simulink model "sdbe_8_11"  (R2012b)
settings: Solver=VariableStepDiscrete  SolverMode=SingleTasking  StartTime=0.0  StopTime=10000  RelTol=1e-3
PreLoadFcn:
  | counter_vals
undefined symbols (not defined in the file or in its folder): sfp
libraries: xbsIndex_r4 x6687, casper_library_misc x35, casper_library_delays x27, dspsigops x16, xps_library x10, r2dbe_vdif_lib x4, r2dbe_adc_lib x3, simulink x1
(part 19 of 58)

== system sdbe_8_11/get_data_from_pkt1/scope ==
  data : Inport
  valid : Inport  Port=2
  Constant : xbsIndex_r4/Constant  const=2  gui_display_data_type=Fixed-point  arith_type=Unsigned  n_bits=7  bin_pt=0  preci_type=Single  exp_width=8  frac_width=24  explicit_period=on  period=1  equ=P=C  opselect=C  inp2=PCIN>>17  opr=+  inp1=P  carry=CIN  dbl_ovrd=off  block_type=constant
  Delay : xbsIndex_r4/Delay  rst=off  infoeditControl=Selection of Reset will increase slice count due to use of real FFs and instead of SRLs  en=off  latency=3  dbl_ovrd=off  reg_retiming=off  block_type=delay
  Delay1 : xbsIndex_r4/Delay  rst=off  infoeditControl=Selection of Reset will increase slice count due to use of real FFs and instead of SRLs  en=off  latency=3  dbl_ovrd=off  reg_retiming=off  block_type=delay
  Disregard Subsystem : xbsIndex_r4/Disregard Subsystem  Tag=discardX  block_type=disregard
  Gateway Out{1..6} (6 alike) : xbsIndex_r4/Gateway Out  inherit_from_input=off  hdl_port=on  timing_constraint=None  locs_specified=off  LOCs={}  UseAsDAC=off  DACChannel='1'  block_type=gatewayout
  Mux : Mux  Inputs=6
  Scope : Scope
      settings: SaveName=ScopeData8
  bus_expand1 : Subsystem  AncestorBlock=casper_library_flow_control/bus_expand  mask(bus_expand){mode=divisions of equal size, outputNum=16, outputWidth=4, outputBinaryPt=0, outputArithmeticType=1, show_format=off, outputToWorkspace=off, variablePrefix=out, outputToModelAsWell=on}
      mask prompts: outputNum "Number of outputs:"; outputWidth "Output width:"; outputBinaryPt "Output binary point position:"; outputArithmeticType "Output arithmetic type (ufix=0, fix=1, bool=2):"; show_format "Print format string?"; outputToWorkspace "Output to workspace?"; variablePrefix "Variable name prefix:"; outputToModelAsWell "Output to model as well?"
      mask help:
      | Expands a 'bus' made using a bus_create or Xilinx
      | concat block.
      | The input will be divided into the specified number
      | of outputs with the specified arithmetic types.
      | Divisions are made from most significant bit.
      mask init: same as sdbe_8_11/get_data_from_pkt/scope/bus_expand1
      settings: AttributesFormatString=16 outputs
      mask TypeOptions mode: divisions of equal size | divisions of arbitrary size
      mask Callback mode: bus_expand_callback();
      mask Callback outputWidth: bus_expand_callback();
      mask Callback outputToWorkspace: bus_expand_callback();
  quant0 : Subsystem
  quant1 : Subsystem
  quant10 : Subsystem
  quant11 : Subsystem
  quant12 : Subsystem
  quant13 : Subsystem
  quant14 : Subsystem
  quant15 : Subsystem
  quant2 : Subsystem
  quant3 : Subsystem
  quant4 : Subsystem
  quant5 : Subsystem
  quant6 : Subsystem
  quant7 : Subsystem
  quant8 : Subsystem
  quant9 : Subsystem
  wires:
  Delay1/1 -> Gateway Out5/1
  Delay/1 -> Gateway Out6/1
  Mux/1 -> Scope/1
  Gateway Out6/1 -> Mux/6
  valid/1 -> Delay/1
  Gateway Out4/1 -> Mux/5
  [p0r_ch3] -> Gateway Out4/1
  Gateway Out3/1 -> Mux/4
  [p0r_ch2] -> Gateway Out3/1
  Gateway Out2/1 -> Mux/3
  [p0r_ch1] -> Gateway Out2/1
  [p0r_ch0] -> Gateway Out1/1
  [p0r_ch0_before] -> Delay1/1
  bus_expand1/7(out10) -> quant6/1(din4)
  bus_expand1/15(out2) -> quant14/1(din4)
  bus_expand1/8(out9) -> quant7/1(din4)
  bus_expand1/13(out4) -> quant12/1(din4)
  bus_expand1/4(out13) -> quant3/1(din4)
  bus_expand1/12(out5) -> quant11/1(din4)
  bus_expand1/10(out7) -> quant9/1(din4)
  bus_expand1/3(out14) -> quant2/1(din4)
  bus_expand1/5(out12) -> quant4/1(din4)
  bus_expand1/1(msb_out16) -> quant0/1(din4), [p0r_ch0_before]
  bus_expand1/11(out6) -> quant10/1(din4)
  bus_expand1/2(out15) -> quant1/1(din4)
  bus_expand1/16(lsb_out1) -> quant15/1(din4)
  bus_expand1/6(out11) -> quant5/1(din4)
  bus_expand1/14(out3) -> quant13/1(din4)
  bus_expand1/9(out8) -> quant8/1(din4)
  Constant/1 -> quant0/2(thr), quant1/2(thr), quant2/2(thr), quant3/2(thr), quant4/2(thr), quant5/2(thr), quant6/2(thr), quant7/2(thr), quant8/2(thr), quant9/2(thr), quant10/2(thr), quant11/2(thr), quant12/2(thr), quant13/2(thr), quant14/2(thr), quant15/2(thr)
  quant0/1(dout2) -> [p0r_ch0]
  quant1/1(dout2) -> [p0i_ch0]
  quant3/1(dout2) -> [p1i_ch0]
  quant2/1(dout2) -> [p1r_ch0]
  quant6/1(dout2) -> [p1r_ch1]
  quant7/1(dout2) -> [p1i_ch1]
  quant4/1(dout2) -> [p0r_ch1]
  quant5/1(dout2) -> [p0i_ch1]
  quant13/1(dout2) -> [p0i_ch3]
  quant14/1(dout2) -> [p1r_ch3]
  quant9/1(dout2) -> [p0i_ch2]
  quant12/1(dout2) -> [p0r_ch3]
  quant11/1(dout2) -> [p1i_ch2]
  quant8/1(dout2) -> [p0r_ch2]
  quant15/1(dout2) -> [p1i_ch3]
  quant10/1(dout2) -> [p1r_ch2]
  Gateway Out1/1 -> Mux/2
  Gateway Out5/1 -> Mux/1
  data/1 -> bus_expand1/1(bus_in)

== system sdbe_8_11/get_data_from_pkt2/gen_valids1 ==
  note: 1 when hdr_val is no and pkt_val is yes
  note: after eof, next high value is hdr
  note: initial value is 0
      |
      | enable on eof
      | send pkt_val through,
      | posedge on output gives hdr_val
      | hdr_val resets to get 0 again, so output is zero
  note: no lat
  note: one lat
  pkt_val : Inport
  eof : Inport  Port=2
  Constant : xbsIndex_r4/Constant  const=1  gui_display_data_type=Boolean  arith_type=Boolean  n_bits=16  bin_pt=14  preci_type=Single  exp_width=8  frac_width=24  explicit_period=off  period=1  equ=P=C  opselect=C  inp2=PCIN>>17  opr=+  inp1=P  carry=CIN  dbl_ovrd=off  block_type=constant
  Constant1 : xbsIndex_r4/Constant  const=1  gui_display_data_type=Boolean  arith_type=Boolean  n_bits=16  bin_pt=14  preci_type=Single  exp_width=8  frac_width=24  explicit_period=off  period=1  equ=P=C  opselect=C  inp2=PCIN>>17  opr=+  inp1=P  carry=CIN  dbl_ovrd=off  block_type=constant
  Delay1 : xbsIndex_r4/Delay  rst=off  infoeditControl=Selection of Reset will increase slice count due to use of real FFs and instead of SRLs  en=off  latency=1  dbl_ovrd=off  reg_retiming=off  block_type=delay
  Delay2 : xbsIndex_r4/Delay  rst=off  infoeditControl=Selection of Reset will increase slice count due to use of real FFs and instead of SRLs  en=off  latency=1  dbl_ovrd=off  reg_retiming=off  block_type=delay
  Logical : xbsIndex_r4/Logical  logical_function=XOR  inputs=2  en=off  latency=0  precision=Full  arith_type=Unsigned  n_bits=16  bin_pt=0  align_bp=on  dbl_ovrd=off  block_type=logical
  Logical1 : xbsIndex_r4/Logical  logical_function=AND  inputs=2  en=off  latency=0  precision=Full  arith_type=Unsigned  n_bits=16  bin_pt=0  align_bp=on  dbl_ovrd=off  block_type=logical
  Register : xbsIndex_r4/Register  init=0  rst=on  en=on  dbl_ovrd=off  block_type=register
  Register1 : xbsIndex_r4/Register  init=0  rst=on  en=on  dbl_ovrd=off  block_type=register
  Register2 : xbsIndex_r4/Register  init=0  rst=off  en=on  dbl_ovrd=off  block_type=register
  posedge : casper_library_misc/posedge  Tag=Rising Edge Detector
  hdr_val : Outport
  data_val : Outport  Port=2
  wires:
  [hdr_val] -> Register1/2
  Constant/1 -> Register1/1
  [hdr_val] -> Register/2
  [pkt_val] -> Delay1/1
  Register1/1 -> Register/3
  pkt_val/1 -> Register/1, [pkt_val]
  eof/1 -> Register2/2, Register1/3
  Register/1 -> posedge/1
  posedge/1 -> Logical/1, hdr_val/1, [hdr_val]
  Logical/1 -> data_val/1
  Logical1/1 -> Logical/2
  Delay1/1 -> Logical1/1
  Constant1/1 -> Register2/1
  Register2/1 -> Delay2/1
  Delay2/1 -> Logical1/2

== system sdbe_8_11/get_data_from_pkt2/npkts ==
  out_reg : Inport
  assert_reg : xbsIndex_r4/Assert  assert_type=on  type_source=Explicitly  gui_display_data_type=Fixed-point  arith_type=Unsigned  n_bits=32  bin_pt=0  preci_type=Single  exp_width=8  frac_width=24  assert_rate=off  rate_source=Explicitly  period=1  output_port=on  block_type=assert
  cast_gw : xbsIndex_r4/Convert  gui_display_data_type=Fixed-point  arith_type=Unsigned  n_bits=32  bin_pt=0  float_type=Single  exp_bits=8  fraction_bits=24  quantization=Truncate  overflow=Wrap  en=off  latency=0  dbl_ovrd=off  pipeline=off  block_type=convert
  io_delay : xbsIndex_r4/Delay  rst=off  infoeditControl=Selection of Reset will increase slice count due to use of real FFs and instead of SRLs  en=off  latency=0  dbl_ovrd=off  reg_retiming=on  block_type=delay
  reint1 : xbsIndex_r4/Reinterpret  force_arith_type=on  arith_type=Unsigned  force_bin_pt=on  bin_pt=0  block_type=reinterpret
  sdbe_8_11_get_data_from_pkt2_npkts_user_data_in : xbsIndex_r4/Gateway Out  inherit_from_input=off  hdl_port=on  timing_constraint=None  locs_specified=off  LOCs={}  UseAsDAC=off  DACChannel='1'  block_type=gatewayout
  sim_out : Outport
  wires:
  io_delay/1 -> cast_gw/1
  cast_gw/1 -> sdbe_8_11_get_data_from_pkt2_npkts_user_data_in/1
  sdbe_8_11_get_data_from_pkt2_npkts_user_data_in/1 -> sim_out/1
  out_reg/1 -> assert_reg/1
  assert_reg/1 -> reint1/1
  reint1/1 -> io_delay/1

== system sdbe_8_11/get_data_from_pkt2/rst ==
  sim_1 : Inport
  io_delay : xbsIndex_r4/Delay  rst=off  infoeditControl=Selection of Reset will increase slice count due to use of real FFs and instead of SRLs  en=off  latency=0  dbl_ovrd=off  reg_retiming=on  block_type=delay
  reint1 : xbsIndex_r4/Reinterpret  force_arith_type=on  arith_type=Unsigned  force_bin_pt=on  bin_pt=0  block_type=reinterpret
  sdbe_8_11_get_data_from_pkt2_rst_user_data_out : xbsIndex_r4/Gateway In  gui_display_data_type=Fixed-point  arith_type=Unsigned  n_bits=32  bin_pt=0  preci_type=Single  exp_width=8  frac_width=24  quantization="Round  (unbiased: +/- Inf)"  overflow=Saturate  period=1  dbl_ovrd=off  timing_constraint=None  locs_specified=off  LOCs={}  UseAsADC=off  ADCChannel='1'  inherit_from_input=off  hdl_port=on  block_type=gatewayin
  slice_reg : xbsIndex_r4/Slice  nbits=32  boolean_output=off  mode=Lower Bit Location + Width  bit1=0  base1=MSB of Input  bit0=0  base0=LSB of Input  dbl_ovrd=off  block_type=slice
  in_reg : Outport
  wires:
  sdbe_8_11_get_data_from_pkt2_rst_user_data_out/1 -> io_delay/1
  sim_1/1 -> sdbe_8_11_get_data_from_pkt2_rst_user_data_out/1
  io_delay/1 -> slice_reg/1
  slice_reg/1 -> reint1/1
  reint1/1 -> in_reg/1

== system sdbe_8_11/get_data_from_pkt2/rx_output ==
  sig : Inport
  val : Inport  Port=2
  eof : Inport  Port=3
  Disregard Subsystem : xbsIndex_r4/Disregard Subsystem  Tag=discardX  block_type=disregard
  Gateway Out : xbsIndex_r4/Gateway Out  inherit_from_input=off  hdl_port=on  timing_constraint=None  locs_specified=off  LOCs={}  UseAsDAC=off  DACChannel='1'  block_type=gatewayout
  Gateway Out1 : xbsIndex_r4/Gateway Out  inherit_from_input=off  hdl_port=on  timing_constraint=None  locs_specified=off  LOCs={}  UseAsDAC=off  DACChannel='1'  block_type=gatewayout
  Gateway Out2 : xbsIndex_r4/Gateway Out  inherit_from_input=off  hdl_port=on  timing_constraint=None  locs_specified=off  LOCs={}  UseAsDAC=off  DACChannel='1'  block_type=gatewayout
  Mux : Mux  Inputs=2
  Scope : Scope  NumInputPorts=2
      settings: YMin=-5~-5  YMax=5~5  SaveName=ScopeData5
  wires:
  sig/1 -> Gateway Out/1
  Gateway Out/1 -> Scope/1  "sig"
  val/1 -> Gateway Out1/1
  eof/1 -> Gateway Out2/1
  Gateway Out2/1 -> Mux/2  "eof"
  Mux/1 -> Scope/2
  Gateway Out1/1 -> Mux/1  "val"

== system sdbe_8_11/get_data_from_pkt2/rx_output1 ==
  hdr : Inport
  hdr_val : Inport  Port=2
  data : Inport  Port=3
  data_val : Inport  Port=4
  Disregard Subsystem : xbsIndex_r4/Disregard Subsystem  Tag=discardX  block_type=disregard
  Gateway Out{,1..3} (4 alike) : xbsIndex_r4/Gateway Out  inherit_from_input=off  hdl_port=on  timing_constraint=None  locs_specified=off  LOCs={}  UseAsDAC=off  DACChannel='1'  block_type=gatewayout
  Mux : Mux  Inputs=2
  Mux1 : Mux  Inputs=2
  Scope : Scope  NumInputPorts=2
      settings: YMin=0~-5  YMax=2.5e+18~5  SaveName=ScopeData5
  wires:
  Mux/1 -> Scope/2  "hdr_val_yellow_data_val_pink"
  data/1 -> Gateway Out2/1
  hdr_val/1 -> Gateway Out1/1
  hdr/1 -> Gateway Out/1
  data_val/1 -> Gateway Out3/1
  Gateway Out3/1 -> Mux/2
  Mux1/1 -> Scope/1  "hdr_yellow_data_pink"
  Gateway Out/1 -> Mux1/1  "sig"
  Gateway Out1/1 -> Mux/1  "val"
  Gateway Out2/1 -> Mux1/2  "eof"

== system sdbe_8_11/get_data_from_pkt2/scope ==
  data : Inport
  valid : Inport  Port=2
  Constant : xbsIndex_r4/Constant  const=2  gui_display_data_type=Fixed-point  arith_type=Unsigned  n_bits=7  bin_pt=0  preci_type=Single  exp_width=8  frac_width=24  explicit_period=on  period=1  equ=P=C  opselect=C  inp2=PCIN>>17  opr=+  inp1=P  carry=CIN  dbl_ovrd=off  block_type=constant
  Delay : xbsIndex_r4/Delay  rst=off  infoeditControl=Selection of Reset will increase slice count due to use of real FFs and instead of SRLs  en=off  latency=3  dbl_ovrd=off  reg_retiming=off  block_type=delay
  Delay1 : xbsIndex_r4/Delay  rst=off  infoeditControl=Selection of Reset will increase slice count due to use of real FFs and instead of SRLs  en=off  latency=3  dbl_ovrd=off  reg_retiming=off  block_type=delay
  Disregard Subsystem : xbsIndex_r4/Disregard Subsystem  Tag=discardX  block_type=disregard
  Gateway Out{1..6} (6 alike) : xbsIndex_r4/Gateway Out  inherit_from_input=off  hdl_port=on  timing_constraint=None  locs_specified=off  LOCs={}  UseAsDAC=off  DACChannel='1'  block_type=gatewayout
  Mux : Mux  Inputs=6
  Scope : Scope
      settings: SaveName=ScopeData8
  bus_expand1 : Subsystem  AncestorBlock=casper_library_flow_control/bus_expand  mask(bus_expand){mode=divisions of equal size, outputNum=16, outputWidth=4, outputBinaryPt=0, outputArithmeticType=1, show_format=off, outputToWorkspace=off, variablePrefix=out, outputToModelAsWell=on}
      mask prompts: outputNum "Number of outputs:"; outputWidth "Output width:"; outputBinaryPt "Output binary point position:"; outputArithmeticType "Output arithmetic type (ufix=0, fix=1, bool=2):"; show_format "Print format string?"; outputToWorkspace "Output to workspace?"; variablePrefix "Variable name prefix:"; outputToModelAsWell "Output to model as well?"
      mask help:
      | Expands a 'bus' made using a bus_create or Xilinx
      | concat block.
      | The input will be divided into the specified number
      | of outputs with the specified arithmetic types.
      | Divisions are made from most significant bit.
      mask init: same as sdbe_8_11/get_data_from_pkt/scope/bus_expand1
      settings: AttributesFormatString=16 outputs
      mask TypeOptions mode: divisions of equal size | divisions of arbitrary size
      mask Callback mode: bus_expand_callback();
      mask Callback outputWidth: bus_expand_callback();
      mask Callback outputToWorkspace: bus_expand_callback();
  quant0 : Subsystem
  quant1 : Subsystem
  quant10 : Subsystem
  quant11 : Subsystem
  quant12 : Subsystem
  quant13 : Subsystem
  quant14 : Subsystem
  quant15 : Subsystem
  quant2 : Subsystem
  quant3 : Subsystem
  quant4 : Subsystem
  quant5 : Subsystem
  quant6 : Subsystem
  quant7 : Subsystem
  quant8 : Subsystem
  quant9 : Subsystem
  wires:
  data/1 -> bus_expand1/1(bus_in)
  Gateway Out5/1 -> Mux/1
  Gateway Out1/1 -> Mux/2
  quant10/1(dout2) -> [p1r_ch2]
  quant15/1(dout2) -> [p1i_ch3]
  quant8/1(dout2) -> [p0r_ch2]
  quant11/1(dout2) -> [p1i_ch2]
  quant12/1(dout2) -> [p0r_ch3]
  quant9/1(dout2) -> [p0i_ch2]
  quant14/1(dout2) -> [p1r_ch3]
  quant13/1(dout2) -> [p0i_ch3]
  quant5/1(dout2) -> [p0i_ch1]
  quant4/1(dout2) -> [p0r_ch1]
  quant7/1(dout2) -> [p1i_ch1]
  quant6/1(dout2) -> [p1r_ch1]
  quant2/1(dout2) -> [p1r_ch0]
  quant3/1(dout2) -> [p1i_ch0]
  quant1/1(dout2) -> [p0i_ch0]
  quant0/1(dout2) -> [p0r_ch0]
  Constant/1 -> quant15/2(thr), quant14/2(thr), quant13/2(thr), quant12/2(thr), quant11/2(thr), quant10/2(thr), quant9/2(thr), quant8/2(thr), quant7/2(thr), quant6/2(thr), quant5/2(thr), quant4/2(thr), quant3/2(thr), quant2/2(thr), quant1/2(thr), quant0/2(thr)
  bus_expand1/9(out8) -> quant8/1(din4)
  bus_expand1/14(out3) -> quant13/1(din4)
  bus_expand1/6(out11) -> quant5/1(din4)
  bus_expand1/16(lsb_out1) -> quant15/1(din4)
  bus_expand1/2(out15) -> quant1/1(din4)
  bus_expand1/11(out6) -> quant10/1(din4)
  bus_expand1/1(msb_out16) -> [p0r_ch0_before], quant0/1(din4)
  bus_expand1/5(out12) -> quant4/1(din4)
  bus_expand1/3(out14) -> quant2/1(din4)
  bus_expand1/10(out7) -> quant9/1(din4)
  bus_expand1/12(out5) -> quant11/1(din4)
  bus_expand1/4(out13) -> quant3/1(din4)
  bus_expand1/13(out4) -> quant12/1(din4)
  bus_expand1/8(out9) -> quant7/1(din4)
  bus_expand1/15(out2) -> quant14/1(din4)
  bus_expand1/7(out10) -> quant6/1(din4)
  [p0r_ch0_before] -> Delay1/1
  [p0r_ch0] -> Gateway Out1/1
  [p0r_ch1] -> Gateway Out2/1
  Gateway Out2/1 -> Mux/3
  [p0r_ch2] -> Gateway Out3/1
  Gateway Out3/1 -> Mux/4
  [p0r_ch3] -> Gateway Out4/1
  Gateway Out4/1 -> Mux/5
  valid/1 -> Delay/1
  Gateway Out6/1 -> Mux/6
  Mux/1 -> Scope/1
  Delay/1 -> Gateway Out6/1
  Delay1/1 -> Gateway Out5/1

== system sdbe_8_11/get_data_from_pkt3/gen_valids1 ==
  note: one lat
  note: no lat
  note: initial value is 0
      |
      | enable on eof
      | send pkt_val through,
      | posedge on output gives hdr_val
      | hdr_val resets to get 0 again, so output is zero
  note: after eof, next high value is hdr
  note: 1 when hdr_val is no and pkt_val is yes
  pkt_val : Inport
  eof : Inport  Port=2
  Constant : xbsIndex_r4/Constant  const=1  gui_display_data_type=Boolean  arith_type=Boolean  n_bits=16  bin_pt=14  preci_type=Single  exp_width=8  frac_width=24  explicit_period=off  period=1  equ=P=C  opselect=C  inp2=PCIN>>17  opr=+  inp1=P  carry=CIN  dbl_ovrd=off  block_type=constant
  Constant1 : xbsIndex_r4/Constant  const=1  gui_display_data_type=Boolean  arith_type=Boolean  n_bits=16  bin_pt=14  preci_type=Single  exp_width=8  frac_width=24  explicit_period=off  period=1  equ=P=C  opselect=C  inp2=PCIN>>17  opr=+  inp1=P  carry=CIN  dbl_ovrd=off  block_type=constant
  Delay1 : xbsIndex_r4/Delay  rst=off  infoeditControl=Selection of Reset will increase slice count due to use of real FFs and instead of SRLs  en=off  latency=1  dbl_ovrd=off  reg_retiming=off  block_type=delay
  Delay2 : xbsIndex_r4/Delay  rst=off  infoeditControl=Selection of Reset will increase slice count due to use of real FFs and instead of SRLs  en=off  latency=1  dbl_ovrd=off  reg_retiming=off  block_type=delay
  Logical : xbsIndex_r4/Logical  logical_function=XOR  inputs=2  en=off  latency=0  precision=Full  arith_type=Unsigned  n_bits=16  bin_pt=0  align_bp=on  dbl_ovrd=off  block_type=logical
  Logical1 : xbsIndex_r4/Logical  logical_function=AND  inputs=2  en=off  latency=0  precision=Full  arith_type=Unsigned  n_bits=16  bin_pt=0  align_bp=on  dbl_ovrd=off  block_type=logical
  Register : xbsIndex_r4/Register  init=0  rst=on  en=on  dbl_ovrd=off  block_type=register
  Register1 : xbsIndex_r4/Register  init=0  rst=on  en=on  dbl_ovrd=off  block_type=register
  Register2 : xbsIndex_r4/Register  init=0  rst=off  en=on  dbl_ovrd=off  block_type=register
  posedge : casper_library_misc/posedge  Tag=Rising Edge Detector
  hdr_val : Outport
  data_val : Outport  Port=2
  wires:
  Delay2/1 -> Logical1/2
  Register2/1 -> Delay2/1
  Constant1/1 -> Register2/1
  Delay1/1 -> Logical1/1
  Logical1/1 -> Logical/2
  Logical/1 -> data_val/1
  posedge/1 -> [hdr_val], hdr_val/1, Logical/1
  Register/1 -> posedge/1
  eof/1 -> Register1/3, Register2/2
  pkt_val/1 -> [pkt_val], Register/1
  Register1/1 -> Register/3
  [pkt_val] -> Delay1/1
  [hdr_val] -> Register/2
  Constant/1 -> Register1/1
  [hdr_val] -> Register1/2

== system sdbe_8_11/get_data_from_pkt3/npkts ==
  out_reg : Inport
  assert_reg : xbsIndex_r4/Assert  assert_type=on  type_source=Explicitly  gui_display_data_type=Fixed-point  arith_type=Unsigned  n_bits=32  bin_pt=0  preci_type=Single  exp_width=8  frac_width=24  assert_rate=off  rate_source=Explicitly  period=1  output_port=on  block_type=assert
  cast_gw : xbsIndex_r4/Convert  gui_display_data_type=Fixed-point  arith_type=Unsigned  n_bits=32  bin_pt=0  float_type=Single  exp_bits=8  fraction_bits=24  quantization=Truncate  overflow=Wrap  en=off  latency=0  dbl_ovrd=off  pipeline=off  block_type=convert
  io_delay : xbsIndex_r4/Delay  rst=off  infoeditControl=Selection of Reset will increase slice count due to use of real FFs and instead of SRLs  en=off  latency=0  dbl_ovrd=off  reg_retiming=on  block_type=delay
  reint1 : xbsIndex_r4/Reinterpret  force_arith_type=on  arith_type=Unsigned  force_bin_pt=on  bin_pt=0  block_type=reinterpret
  sdbe_8_11_get_data_from_pkt3_npkts_user_data_in : xbsIndex_r4/Gateway Out  inherit_from_input=off  hdl_port=on  timing_constraint=None  locs_specified=off  LOCs={}  UseAsDAC=off  DACChannel='1'  block_type=gatewayout
  sim_out : Outport
  wires:
  io_delay/1 -> cast_gw/1
  cast_gw/1 -> sdbe_8_11_get_data_from_pkt3_npkts_user_data_in/1
  sdbe_8_11_get_data_from_pkt3_npkts_user_data_in/1 -> sim_out/1
  out_reg/1 -> assert_reg/1
  assert_reg/1 -> reint1/1
  reint1/1 -> io_delay/1

== system sdbe_8_11/get_data_from_pkt3/rst ==
  sim_1 : Inport
  io_delay : xbsIndex_r4/Delay  rst=off  infoeditControl=Selection of Reset will increase slice count due to use of real FFs and instead of SRLs  en=off  latency=0  dbl_ovrd=off  reg_retiming=on  block_type=delay
  reint1 : xbsIndex_r4/Reinterpret  force_arith_type=on  arith_type=Unsigned  force_bin_pt=on  bin_pt=0  block_type=reinterpret
  sdbe_8_11_get_data_from_pkt3_rst_user_data_out : xbsIndex_r4/Gateway In  gui_display_data_type=Fixed-point  arith_type=Unsigned  n_bits=32  bin_pt=0  preci_type=Single  exp_width=8  frac_width=24  quantization="Round  (unbiased: +/- Inf)"  overflow=Saturate  period=1  dbl_ovrd=off  timing_constraint=None  locs_specified=off  LOCs={}  UseAsADC=off  ADCChannel='1'  inherit_from_input=off  hdl_port=on  block_type=gatewayin
  slice_reg : xbsIndex_r4/Slice  nbits=32  boolean_output=off  mode=Lower Bit Location + Width  bit1=0  base1=MSB of Input  bit0=0  base0=LSB of Input  dbl_ovrd=off  block_type=slice
  in_reg : Outport
  wires:
  sdbe_8_11_get_data_from_pkt3_rst_user_data_out/1 -> io_delay/1
  sim_1/1 -> sdbe_8_11_get_data_from_pkt3_rst_user_data_out/1
  io_delay/1 -> slice_reg/1
  slice_reg/1 -> reint1/1
  reint1/1 -> in_reg/1

== system sdbe_8_11/get_data_from_pkt3/rx_output ==
  sig : Inport
  val : Inport  Port=2
  eof : Inport  Port=3
  Disregard Subsystem : xbsIndex_r4/Disregard Subsystem  Tag=discardX  block_type=disregard
  Gateway Out : xbsIndex_r4/Gateway Out  inherit_from_input=off  hdl_port=on  timing_constraint=None  locs_specified=off  LOCs={}  UseAsDAC=off  DACChannel='1'  block_type=gatewayout
  Gateway Out1 : xbsIndex_r4/Gateway Out  inherit_from_input=off  hdl_port=on  timing_constraint=None  locs_specified=off  LOCs={}  UseAsDAC=off  DACChannel='1'  block_type=gatewayout
  Gateway Out2 : xbsIndex_r4/Gateway Out  inherit_from_input=off  hdl_port=on  timing_constraint=None  locs_specified=off  LOCs={}  UseAsDAC=off  DACChannel='1'  block_type=gatewayout
  Mux : Mux  Inputs=2
  Scope : Scope  NumInputPorts=2
      settings: YMin=-5~-5  YMax=5~5  SaveName=ScopeData5
  wires:
  Gateway Out1/1 -> Mux/1  "val"
  Mux/1 -> Scope/2
  Gateway Out2/1 -> Mux/2  "eof"
  eof/1 -> Gateway Out2/1
  val/1 -> Gateway Out1/1
  Gateway Out/1 -> Scope/1  "sig"
  sig/1 -> Gateway Out/1

== system sdbe_8_11/get_data_from_pkt3/rx_output1 ==
  hdr : Inport
  hdr_val : Inport  Port=2
  data : Inport  Port=3
  data_val : Inport  Port=4
  Disregard Subsystem : xbsIndex_r4/Disregard Subsystem  Tag=discardX  block_type=disregard
  Gateway Out{,1..3} (4 alike) : xbsIndex_r4/Gateway Out  inherit_from_input=off  hdl_port=on  timing_constraint=None  locs_specified=off  LOCs={}  UseAsDAC=off  DACChannel='1'  block_type=gatewayout
  Mux : Mux  Inputs=2
  Mux1 : Mux  Inputs=2
  Scope : Scope  NumInputPorts=2
      settings: YMin=0~-5  YMax=2.5e+18~5  SaveName=ScopeData5
  wires:
  Gateway Out2/1 -> Mux1/2  "eof"
  Gateway Out1/1 -> Mux/1  "val"
  Gateway Out/1 -> Mux1/1  "sig"
  Mux1/1 -> Scope/1  "hdr_yellow_data_pink"
  Gateway Out3/1 -> Mux/2
  data_val/1 -> Gateway Out3/1
  hdr/1 -> Gateway Out/1
  hdr_val/1 -> Gateway Out1/1
  data/1 -> Gateway Out2/1
  Mux/1 -> Scope/2  "hdr_val_yellow_data_val_pink"

== system sdbe_8_11/get_data_from_pkt3/scope ==
  data : Inport
  valid : Inport  Port=2
  Constant : xbsIndex_r4/Constant  const=2  gui_display_data_type=Fixed-point  arith_type=Unsigned  n_bits=7  bin_pt=0  preci_type=Single  exp_width=8  frac_width=24  explicit_period=on  period=1  equ=P=C  opselect=C  inp2=PCIN>>17  opr=+  inp1=P  carry=CIN  dbl_ovrd=off  block_type=constant
  Delay : xbsIndex_r4/Delay  rst=off  infoeditControl=Selection of Reset will increase slice count due to use of real FFs and instead of SRLs  en=off  latency=3  dbl_ovrd=off  reg_retiming=off  block_type=delay
  Delay1 : xbsIndex_r4/Delay  rst=off  infoeditControl=Selection of Reset will increase slice count due to use of real FFs and instead of SRLs  en=off  latency=3  dbl_ovrd=off  reg_retiming=off  block_type=delay
  Disregard Subsystem : xbsIndex_r4/Disregard Subsystem  Tag=discardX  block_type=disregard
  Gateway Out{1..6} (6 alike) : xbsIndex_r4/Gateway Out  inherit_from_input=off  hdl_port=on  timing_constraint=None  locs_specified=off  LOCs={}  UseAsDAC=off  DACChannel='1'  block_type=gatewayout
  Mux : Mux  Inputs=6
  Scope : Scope
      settings: SaveName=ScopeData8
  bus_expand1 : Subsystem  AncestorBlock=casper_library_flow_control/bus_expand  mask(bus_expand){mode=divisions of equal size, outputNum=16, outputWidth=4, outputBinaryPt=0, outputArithmeticType=1, show_format=off, outputToWorkspace=off, variablePrefix=out, outputToModelAsWell=on}
      mask prompts: outputNum "Number of outputs:"; outputWidth "Output width:"; outputBinaryPt "Output binary point position:"; outputArithmeticType "Output arithmetic type (ufix=0, fix=1, bool=2):"; show_format "Print format string?"; outputToWorkspace "Output to workspace?"; variablePrefix "Variable name prefix:"; outputToModelAsWell "Output to model as well?"
      mask help:
      | Expands a 'bus' made using a bus_create or Xilinx
      | concat block.
      | The input will be divided into the specified number
      | of outputs with the specified arithmetic types.
      | Divisions are made from most significant bit.
      mask init: same as sdbe_8_11/get_data_from_pkt/scope/bus_expand1
      settings: AttributesFormatString=16 outputs
      mask TypeOptions mode: divisions of equal size | divisions of arbitrary size
      mask Callback mode: bus_expand_callback();
      mask Callback outputWidth: bus_expand_callback();
      mask Callback outputToWorkspace: bus_expand_callback();
  quant0 : Subsystem
  quant1 : Subsystem
  quant10 : Subsystem
  quant11 : Subsystem
  quant12 : Subsystem
  quant13 : Subsystem
  quant14 : Subsystem
  quant15 : Subsystem
  quant2 : Subsystem
  quant3 : Subsystem
  quant4 : Subsystem
  quant5 : Subsystem
  quant6 : Subsystem
  quant7 : Subsystem
  quant8 : Subsystem
  quant9 : Subsystem
  wires:
  Delay1/1 -> Gateway Out5/1
  Delay/1 -> Gateway Out6/1
  Mux/1 -> Scope/1
  Gateway Out6/1 -> Mux/6
  valid/1 -> Delay/1
  Gateway Out4/1 -> Mux/5
  [p0r_ch3] -> Gateway Out4/1
  Gateway Out3/1 -> Mux/4
  [p0r_ch2] -> Gateway Out3/1
  Gateway Out2/1 -> Mux/3
  [p0r_ch1] -> Gateway Out2/1
  [p0r_ch0] -> Gateway Out1/1
  [p0r_ch0_before] -> Delay1/1
  bus_expand1/7(out10) -> quant6/1(din4)
  bus_expand1/15(out2) -> quant14/1(din4)
  bus_expand1/8(out9) -> quant7/1(din4)
  bus_expand1/13(out4) -> quant12/1(din4)
  bus_expand1/4(out13) -> quant3/1(din4)
  bus_expand1/12(out5) -> quant11/1(din4)
  bus_expand1/10(out7) -> quant9/1(din4)
  bus_expand1/3(out14) -> quant2/1(din4)
  bus_expand1/5(out12) -> quant4/1(din4)
  bus_expand1/1(msb_out16) -> quant0/1(din4), [p0r_ch0_before]
  bus_expand1/11(out6) -> quant10/1(din4)
  bus_expand1/2(out15) -> quant1/1(din4)
  bus_expand1/16(lsb_out1) -> quant15/1(din4)
  bus_expand1/6(out11) -> quant5/1(din4)
  bus_expand1/14(out3) -> quant13/1(din4)
  bus_expand1/9(out8) -> quant8/1(din4)
  Constant/1 -> quant0/2(thr), quant1/2(thr), quant2/2(thr), quant3/2(thr), quant4/2(thr), quant5/2(thr), quant6/2(thr), quant7/2(thr), quant8/2(thr), quant9/2(thr), quant10/2(thr), quant11/2(thr), quant12/2(thr), quant13/2(thr), quant14/2(thr), quant15/2(thr)
  quant0/1(dout2) -> [p0r_ch0]
  quant1/1(dout2) -> [p0i_ch0]
  quant3/1(dout2) -> [p1i_ch0]
  quant2/1(dout2) -> [p1r_ch0]
  quant6/1(dout2) -> [p1r_ch1]
  quant7/1(dout2) -> [p1i_ch1]
  quant4/1(dout2) -> [p0r_ch1]
  quant5/1(dout2) -> [p0i_ch1]
  quant13/1(dout2) -> [p0i_ch3]
  quant14/1(dout2) -> [p1r_ch3]
  quant9/1(dout2) -> [p0i_ch2]
  quant12/1(dout2) -> [p0r_ch3]
  quant11/1(dout2) -> [p1i_ch2]
  quant8/1(dout2) -> [p0r_ch2]
  quant15/1(dout2) -> [p1i_ch3]
  quant10/1(dout2) -> [p1r_ch2]
  Gateway Out1/1 -> Mux/2
  Gateway Out5/1 -> Mux/1
  data/1 -> bus_expand1/1(bus_in)

== system sdbe_8_11/network_buffer/er ==
  out_reg : Inport
  assert_reg : xbsIndex_r4/Assert  assert_type=on  type_source=Explicitly  gui_display_data_type=Fixed-point  arith_type=Unsigned  n_bits=32  bin_pt=0  preci_type=Single  exp_width=8  frac_width=24  assert_rate=off  rate_source=Explicitly  period=1  output_port=on  block_type=assert
  cast_gw : xbsIndex_r4/Convert  gui_display_data_type=Fixed-point  arith_type=Unsigned  n_bits=32  bin_pt=0  float_type=Single  exp_bits=8  fraction_bits=24  quantization=Truncate  overflow=Wrap  en=off  latency=0  dbl_ovrd=off  pipeline=off  block_type=convert
  io_delay : xbsIndex_r4/Delay  rst=off  infoeditControl=Selection of Reset will increase slice count due to use of real FFs and instead of SRLs  en=off  latency=0  dbl_ovrd=off  reg_retiming=on  block_type=delay
  reint1 : xbsIndex_r4/Reinterpret  force_arith_type=on  arith_type=Unsigned  force_bin_pt=on  bin_pt=0  block_type=reinterpret
  sdbe_8_11_network_buffer_er_user_data_in : xbsIndex_r4/Gateway Out  inherit_from_input=off  hdl_port=on  timing_constraint=None  locs_specified=off  LOCs={}  UseAsDAC=off  DACChannel='1'  block_type=gatewayout
  sim_out : Outport
  wires:
  io_delay/1 -> cast_gw/1
  cast_gw/1 -> sdbe_8_11_network_buffer_er_user_data_in/1
  sdbe_8_11_network_buffer_er_user_data_in/1 -> sim_out/1
  out_reg/1 -> assert_reg/1
  assert_reg/1 -> reint1/1
  reint1/1 -> io_delay/1

== system sdbe_8_11/network_buffer/ew ==
  out_reg : Inport
  assert_reg : xbsIndex_r4/Assert  assert_type=on  type_source=Explicitly  gui_display_data_type=Fixed-point  arith_type=Unsigned  n_bits=32  bin_pt=0  preci_type=Single  exp_width=8  frac_width=24  assert_rate=off  rate_source=Explicitly  period=1  output_port=on  block_type=assert
  cast_gw : xbsIndex_r4/Convert  gui_display_data_type=Fixed-point  arith_type=Unsigned  n_bits=32  bin_pt=0  float_type=Single  exp_bits=8  fraction_bits=24  quantization=Truncate  overflow=Wrap  en=off  latency=0  dbl_ovrd=off  pipeline=off  block_type=convert
  io_delay : xbsIndex_r4/Delay  rst=off  infoeditControl=Selection of Reset will increase slice count due to use of real FFs and instead of SRLs  en=off  latency=0  dbl_ovrd=off  reg_retiming=on  block_type=delay
  reint1 : xbsIndex_r4/Reinterpret  force_arith_type=on  arith_type=Unsigned  force_bin_pt=on  bin_pt=0  block_type=reinterpret
  sdbe_8_11_network_buffer_ew_user_data_in : xbsIndex_r4/Gateway Out  inherit_from_input=off  hdl_port=on  timing_constraint=None  locs_specified=off  LOCs={}  UseAsDAC=off  DACChannel='1'  block_type=gatewayout
  sim_out : Outport
  wires:
  io_delay/1 -> cast_gw/1
  cast_gw/1 -> sdbe_8_11_network_buffer_ew_user_data_in/1
  sdbe_8_11_network_buffer_ew_user_data_in/1 -> sim_out/1
  out_reg/1 -> assert_reg/1
  assert_reg/1 -> reint1/1
  reint1/1 -> io_delay/1

== system sdbe_8_11/network_buffer/ext_257 ==
  in : Inport
  Delay : xbsIndex_r4/Delay  rst=off  infoeditControl=Selection of Reset will increase slice count due to use of real FFs and instead of SRLs  en=off  latency=1  dbl_ovrd=off  reg_retiming=off  block_type=delay
  Delay1 : xbsIndex_r4/Delay  rst=off  infoeditControl=Selection of Reset will increase slice count due to use of real FFs and instead of SRLs  en=off  latency=2  dbl_ovrd=off  reg_retiming=off  block_type=delay
  Delay2 : xbsIndex_r4/Delay  rst=off  infoeditControl=Selection of Reset will increase slice count due to use of real FFs and instead of SRLs  en=off  latency=4  dbl_ovrd=off  reg_retiming=off  block_type=delay
  Delay3 : xbsIndex_r4/Delay  rst=off  infoeditControl=Selection of Reset will increase slice count due to use of real FFs and instead of SRLs  en=off  latency=8  dbl_ovrd=off  reg_retiming=off  block_type=delay
  Delay4 : xbsIndex_r4/Delay  rst=off  infoeditControl=Selection of Reset will increase slice count due to use of real FFs and instead of SRLs  en=off  latency=16  dbl_ovrd=off  reg_retiming=off  block_type=delay
  Delay5 : xbsIndex_r4/Delay  rst=off  infoeditControl=Selection of Reset will increase slice count due to use of real FFs and instead of SRLs  en=off  latency=32  dbl_ovrd=off  reg_retiming=off  block_type=delay
  Delay6 : xbsIndex_r4/Delay  rst=off  infoeditControl=Selection of Reset will increase slice count due to use of real FFs and instead of SRLs  en=off  latency=64  dbl_ovrd=off  reg_retiming=off  block_type=delay
  Delay7 : xbsIndex_r4/Delay  rst=off  infoeditControl=Selection of Reset will increase slice count due to use of real FFs and instead of SRLs  en=off  latency=128  dbl_ovrd=off  reg_retiming=off  block_type=delay
  Delay8 : xbsIndex_r4/Delay  rst=off  infoeditControl=Selection of Reset will increase slice count due to use of real FFs and instead of SRLs  en=off  latency=1  dbl_ovrd=off  reg_retiming=off  block_type=delay
  Logical{,1..8} (9 alike) : xbsIndex_r4/Logical  logical_function=OR  inputs=2  en=off  latency=0  precision=Full  arith_type=Unsigned  n_bits=16  bin_pt=0  align_bp=on  dbl_ovrd=off  block_type=logical
  out : Outport
  wires:
  Delay/1 -> Logical/2
  in/1 -> Delay/1, Logical/1
  Delay1/1 -> Logical1/2
  Logical/1 -> Delay1/1, Logical1/1
  Delay2/1 -> Logical2/2
  Logical1/1 -> Delay2/1, Logical2/1
  Logical2/1 -> Delay3/1, Logical3/1
  Logical3/1 -> Delay4/1, Logical4/1
  Logical4/1 -> Delay5/1, Logical5/1
  Logical5/1 -> Delay6/1, Logical6/1
  Delay3/1 -> Logical3/2
  Delay4/1 -> Logical4/2
  Delay6/1 -> Logical6/2
  Delay5/1 -> Logical5/2
  Logical6/1 -> Logical7/1, Delay7/1
  Delay7/1 -> Logical7/2
  Delay8/1 -> Logical8/2
  Logical8/1 -> out/1
  Logical7/1 -> Delay8/1, Logical8/1

== system sdbe_8_11/network_buffer/fr ==
  out_reg : Inport
  assert_reg : xbsIndex_r4/Assert  assert_type=on  type_source=Explicitly  gui_display_data_type=Fixed-point  arith_type=Unsigned  n_bits=32  bin_pt=0  preci_type=Single  exp_width=8  frac_width=24  assert_rate=off  rate_source=Explicitly  period=1  output_port=on  block_type=assert
  cast_gw : xbsIndex_r4/Convert  gui_display_data_type=Fixed-point  arith_type=Unsigned  n_bits=32  bin_pt=0  float_type=Single  exp_bits=8  fraction_bits=24  quantization=Truncate  overflow=Wrap  en=off  latency=0  dbl_ovrd=off  pipeline=off  block_type=convert
  io_delay : xbsIndex_r4/Delay  rst=off  infoeditControl=Selection of Reset will increase slice count due to use of real FFs and instead of SRLs  en=off  latency=0  dbl_ovrd=off  reg_retiming=on  block_type=delay
  reint1 : xbsIndex_r4/Reinterpret  force_arith_type=on  arith_type=Unsigned  force_bin_pt=on  bin_pt=0  block_type=reinterpret
  sdbe_8_11_network_buffer_fr_user_data_in : xbsIndex_r4/Gateway Out  inherit_from_input=off  hdl_port=on  timing_constraint=None  locs_specified=off  LOCs={}  UseAsDAC=off  DACChannel='1'  block_type=gatewayout
  sim_out : Outport
  wires:
  io_delay/1 -> cast_gw/1
  cast_gw/1 -> sdbe_8_11_network_buffer_fr_user_data_in/1
  sdbe_8_11_network_buffer_fr_user_data_in/1 -> sim_out/1
  out_reg/1 -> assert_reg/1
  assert_reg/1 -> reint1/1
  reint1/1 -> io_delay/1

== system sdbe_8_11/network_buffer/full ==
  out_reg : Inport
  assert_reg : xbsIndex_r4/Assert  assert_type=on  type_source=Explicitly  gui_display_data_type=Fixed-point  arith_type=Unsigned  n_bits=32  bin_pt=0  preci_type=Single  exp_width=8  frac_width=24  assert_rate=off  rate_source=Explicitly  period=1  output_port=on  block_type=assert
  cast_gw : xbsIndex_r4/Convert  gui_display_data_type=Fixed-point  arith_type=Unsigned  n_bits=32  bin_pt=0  float_type=Single  exp_bits=8  fraction_bits=24  quantization=Truncate  overflow=Wrap  en=off  latency=0  dbl_ovrd=off  pipeline=off  block_type=convert
  io_delay : xbsIndex_r4/Delay  rst=off  infoeditControl=Selection of Reset will increase slice count due to use of real FFs and instead of SRLs  en=off  latency=0  dbl_ovrd=off  reg_retiming=on  block_type=delay
  reint1 : xbsIndex_r4/Reinterpret  force_arith_type=on  arith_type=Unsigned  force_bin_pt=on  bin_pt=0  block_type=reinterpret
  sdbe_8_11_network_buffer_full_user_data_in : xbsIndex_r4/Gateway Out  inherit_from_input=off  hdl_port=on  timing_constraint=None  locs_specified=off  LOCs={}  UseAsDAC=off  DACChannel='1'  block_type=gatewayout
  sim_out : Outport
  wires:
  io_delay/1 -> cast_gw/1
  cast_gw/1 -> sdbe_8_11_network_buffer_full_user_data_in/1
  sdbe_8_11_network_buffer_full_user_data_in/1 -> sim_out/1
  out_reg/1 -> assert_reg/1
  assert_reg/1 -> reint1/1
  reint1/1 -> io_delay/1

== system sdbe_8_11/network_buffer/fw ==
  out_reg : Inport
  assert_reg : xbsIndex_r4/Assert  assert_type=on  type_source=Explicitly  gui_display_data_type=Fixed-point  arith_type=Unsigned  n_bits=32  bin_pt=0  preci_type=Single  exp_width=8  frac_width=24  assert_rate=off  rate_source=Explicitly  period=1  output_port=on  block_type=assert
  cast_gw : xbsIndex_r4/Convert  gui_display_data_type=Fixed-point  arith_type=Unsigned  n_bits=32  bin_pt=0  float_type=Single  exp_bits=8  fraction_bits=24  quantization=Truncate  overflow=Wrap  en=off  latency=0  dbl_ovrd=off  pipeline=off  block_type=convert
  io_delay : xbsIndex_r4/Delay  rst=off  infoeditControl=Selection of Reset will increase slice count due to use of real FFs and instead of SRLs  en=off  latency=0  dbl_ovrd=off  reg_retiming=on  block_type=delay
  reint1 : xbsIndex_r4/Reinterpret  force_arith_type=on  arith_type=Unsigned  force_bin_pt=on  bin_pt=0  block_type=reinterpret
  sdbe_8_11_network_buffer_fw_user_data_in : xbsIndex_r4/Gateway Out  inherit_from_input=off  hdl_port=on  timing_constraint=None  locs_specified=off  LOCs={}  UseAsDAC=off  DACChannel='1'  block_type=gatewayout
  sim_out : Outport
  wires:
  io_delay/1 -> cast_gw/1
  cast_gw/1 -> sdbe_8_11_network_buffer_fw_user_data_in/1
  sdbe_8_11_network_buffer_fw_user_data_in/1 -> sim_out/1
  out_reg/1 -> assert_reg/1
  assert_reg/1 -> reint1/1
  reint1/1 -> io_delay/1

== system sdbe_8_11/network_buffer1/er ==
  out_reg : Inport
  assert_reg : xbsIndex_r4/Assert  assert_type=on  type_source=Explicitly  gui_display_data_type=Fixed-point  arith_type=Unsigned  n_bits=32  bin_pt=0  preci_type=Single  exp_width=8  frac_width=24  assert_rate=off  rate_source=Explicitly  period=1  output_port=on  block_type=assert
  cast_gw : xbsIndex_r4/Convert  gui_display_data_type=Fixed-point  arith_type=Unsigned  n_bits=32  bin_pt=0  float_type=Single  exp_bits=8  fraction_bits=24  quantization=Truncate  overflow=Wrap  en=off  latency=0  dbl_ovrd=off  pipeline=off  block_type=convert
  io_delay : xbsIndex_r4/Delay  rst=off  infoeditControl=Selection of Reset will increase slice count due to use of real FFs and instead of SRLs  en=off  latency=0  dbl_ovrd=off  reg_retiming=on  block_type=delay
  reint1 : xbsIndex_r4/Reinterpret  force_arith_type=on  arith_type=Unsigned  force_bin_pt=on  bin_pt=0  block_type=reinterpret
  sdbe_8_11_network_buffer1_er_user_data_in : xbsIndex_r4/Gateway Out  inherit_from_input=off  hdl_port=on  timing_constraint=None  locs_specified=off  LOCs={}  UseAsDAC=off  DACChannel='1'  block_type=gatewayout
  sim_out : Outport
  wires:
  io_delay/1 -> cast_gw/1
  cast_gw/1 -> sdbe_8_11_network_buffer1_er_user_data_in/1
  sdbe_8_11_network_buffer1_er_user_data_in/1 -> sim_out/1
  out_reg/1 -> assert_reg/1
  assert_reg/1 -> reint1/1
  reint1/1 -> io_delay/1

== system sdbe_8_11/network_buffer1/ew ==
  out_reg : Inport
  assert_reg : xbsIndex_r4/Assert  assert_type=on  type_source=Explicitly  gui_display_data_type=Fixed-point  arith_type=Unsigned  n_bits=32  bin_pt=0  preci_type=Single  exp_width=8  frac_width=24  assert_rate=off  rate_source=Explicitly  period=1  output_port=on  block_type=assert
  cast_gw : xbsIndex_r4/Convert  gui_display_data_type=Fixed-point  arith_type=Unsigned  n_bits=32  bin_pt=0  float_type=Single  exp_bits=8  fraction_bits=24  quantization=Truncate  overflow=Wrap  en=off  latency=0  dbl_ovrd=off  pipeline=off  block_type=convert
  io_delay : xbsIndex_r4/Delay  rst=off  infoeditControl=Selection of Reset will increase slice count due to use of real FFs and instead of SRLs  en=off  latency=0  dbl_ovrd=off  reg_retiming=on  block_type=delay
  reint1 : xbsIndex_r4/Reinterpret  force_arith_type=on  arith_type=Unsigned  force_bin_pt=on  bin_pt=0  block_type=reinterpret
  sdbe_8_11_network_buffer1_ew_user_data_in : xbsIndex_r4/Gateway Out  inherit_from_input=off  hdl_port=on  timing_constraint=None  locs_specified=off  LOCs={}  UseAsDAC=off  DACChannel='1'  block_type=gatewayout
  sim_out : Outport
  wires:
  io_delay/1 -> cast_gw/1
  cast_gw/1 -> sdbe_8_11_network_buffer1_ew_user_data_in/1
  sdbe_8_11_network_buffer1_ew_user_data_in/1 -> sim_out/1
  out_reg/1 -> assert_reg/1
  assert_reg/1 -> reint1/1
  reint1/1 -> io_delay/1

== system sdbe_8_11/network_buffer1/ext_257 ==
  in : Inport
  Delay : xbsIndex_r4/Delay  rst=off  infoeditControl=Selection of Reset will increase slice count due to use of real FFs and instead of SRLs  en=off  latency=1  dbl_ovrd=off  reg_retiming=off  block_type=delay
  Delay1 : xbsIndex_r4/Delay  rst=off  infoeditControl=Selection of Reset will increase slice count due to use of real FFs and instead of SRLs  en=off  latency=2  dbl_ovrd=off  reg_retiming=off  block_type=delay
  Delay2 : xbsIndex_r4/Delay  rst=off  infoeditControl=Selection of Reset will increase slice count due to use of real FFs and instead of SRLs  en=off  latency=4  dbl_ovrd=off  reg_retiming=off  block_type=delay
  Delay3 : xbsIndex_r4/Delay  rst=off  infoeditControl=Selection of Reset will increase slice count due to use of real FFs and instead of SRLs  en=off  latency=8  dbl_ovrd=off  reg_retiming=off  block_type=delay
  Delay4 : xbsIndex_r4/Delay  rst=off  infoeditControl=Selection of Reset will increase slice count due to use of real FFs and instead of SRLs  en=off  latency=16  dbl_ovrd=off  reg_retiming=off  block_type=delay
  Delay5 : xbsIndex_r4/Delay  rst=off  infoeditControl=Selection of Reset will increase slice count due to use of real FFs and instead of SRLs  en=off  latency=32  dbl_ovrd=off  reg_retiming=off  block_type=delay
  Delay6 : xbsIndex_r4/Delay  rst=off  infoeditControl=Selection of Reset will increase slice count due to use of real FFs and instead of SRLs  en=off  latency=64  dbl_ovrd=off  reg_retiming=off  block_type=delay
  Delay7 : xbsIndex_r4/Delay  rst=off  infoeditControl=Selection of Reset will increase slice count due to use of real FFs and instead of SRLs  en=off  latency=128  dbl_ovrd=off  reg_retiming=off  block_type=delay
  Delay8 : xbsIndex_r4/Delay  rst=off  infoeditControl=Selection of Reset will increase slice count due to use of real FFs and instead of SRLs  en=off  latency=1  dbl_ovrd=off  reg_retiming=off  block_type=delay
  Logical{,1..8} (9 alike) : xbsIndex_r4/Logical  logical_function=OR  inputs=2  en=off  latency=0  precision=Full  arith_type=Unsigned  n_bits=16  bin_pt=0  align_bp=on  dbl_ovrd=off  block_type=logical
  out : Outport
  wires:
  Logical7/1 -> Logical8/1, Delay8/1
  Logical8/1 -> out/1
  Delay8/1 -> Logical8/2
  Delay7/1 -> Logical7/2
  Logical6/1 -> Delay7/1, Logical7/1
  Delay5/1 -> Logical5/2
  Delay6/1 -> Logical6/2
  Delay4/1 -> Logical4/2
  Delay3/1 -> Logical3/2
  Logical5/1 -> Logical6/1, Delay6/1
  Logical4/1 -> Logical5/1, Delay5/1
  Logical3/1 -> Logical4/1, Delay4/1
  Logical2/1 -> Logical3/1, Delay3/1
  Logical1/1 -> Logical2/1, Delay2/1
  Delay2/1 -> Logical2/2
  Logical/1 -> Logical1/1, Delay1/1
  Delay1/1 -> Logical1/2
  in/1 -> Logical/1, Delay/1
  Delay/1 -> Logical/2

== system sdbe_8_11/network_buffer1/fr ==
  out_reg : Inport
  assert_reg : xbsIndex_r4/Assert  assert_type=on  type_source=Explicitly  gui_display_data_type=Fixed-point  arith_type=Unsigned  n_bits=32  bin_pt=0  preci_type=Single  exp_width=8  frac_width=24  assert_rate=off  rate_source=Explicitly  period=1  output_port=on  block_type=assert
  cast_gw : xbsIndex_r4/Convert  gui_display_data_type=Fixed-point  arith_type=Unsigned  n_bits=32  bin_pt=0  float_type=Single  exp_bits=8  fraction_bits=24  quantization=Truncate  overflow=Wrap  en=off  latency=0  dbl_ovrd=off  pipeline=off  block_type=convert
  io_delay : xbsIndex_r4/Delay  rst=off  infoeditControl=Selection of Reset will increase slice count due to use of real FFs and instead of SRLs  en=off  latency=0  dbl_ovrd=off  reg_retiming=on  block_type=delay
  reint1 : xbsIndex_r4/Reinterpret  force_arith_type=on  arith_type=Unsigned  force_bin_pt=on  bin_pt=0  block_type=reinterpret
  sdbe_8_11_network_buffer1_fr_user_data_in : xbsIndex_r4/Gateway Out  inherit_from_input=off  hdl_port=on  timing_constraint=None  locs_specified=off  LOCs={}  UseAsDAC=off  DACChannel='1'  block_type=gatewayout
  sim_out : Outport
  wires:
  io_delay/1 -> cast_gw/1
  cast_gw/1 -> sdbe_8_11_network_buffer1_fr_user_data_in/1
  sdbe_8_11_network_buffer1_fr_user_data_in/1 -> sim_out/1
  out_reg/1 -> assert_reg/1
  assert_reg/1 -> reint1/1
  reint1/1 -> io_delay/1

== system sdbe_8_11/network_buffer1/full ==
  out_reg : Inport
  assert_reg : xbsIndex_r4/Assert  assert_type=on  type_source=Explicitly  gui_display_data_type=Fixed-point  arith_type=Unsigned  n_bits=32  bin_pt=0  preci_type=Single  exp_width=8  frac_width=24  assert_rate=off  rate_source=Explicitly  period=1  output_port=on  block_type=assert
  cast_gw : xbsIndex_r4/Convert  gui_display_data_type=Fixed-point  arith_type=Unsigned  n_bits=32  bin_pt=0  float_type=Single  exp_bits=8  fraction_bits=24  quantization=Truncate  overflow=Wrap  en=off  latency=0  dbl_ovrd=off  pipeline=off  block_type=convert
  io_delay : xbsIndex_r4/Delay  rst=off  infoeditControl=Selection of Reset will increase slice count due to use of real FFs and instead of SRLs  en=off  latency=0  dbl_ovrd=off  reg_retiming=on  block_type=delay
  reint1 : xbsIndex_r4/Reinterpret  force_arith_type=on  arith_type=Unsigned  force_bin_pt=on  bin_pt=0  block_type=reinterpret
  sdbe_8_11_network_buffer1_full_user_data_in : xbsIndex_r4/Gateway Out  inherit_from_input=off  hdl_port=on  timing_constraint=None  locs_specified=off  LOCs={}  UseAsDAC=off  DACChannel='1'  block_type=gatewayout
  sim_out : Outport
  wires:
  io_delay/1 -> cast_gw/1
  cast_gw/1 -> sdbe_8_11_network_buffer1_full_user_data_in/1
  sdbe_8_11_network_buffer1_full_user_data_in/1 -> sim_out/1
  out_reg/1 -> assert_reg/1
  assert_reg/1 -> reint1/1
  reint1/1 -> io_delay/1

== system sdbe_8_11/network_buffer1/fw ==
  out_reg : Inport
  assert_reg : xbsIndex_r4/Assert  assert_type=on  type_source=Explicitly  gui_display_data_type=Fixed-point  arith_type=Unsigned  n_bits=32  bin_pt=0  preci_type=Single  exp_width=8  frac_width=24  assert_rate=off  rate_source=Explicitly  period=1  output_port=on  block_type=assert
  cast_gw : xbsIndex_r4/Convert  gui_display_data_type=Fixed-point  arith_type=Unsigned  n_bits=32  bin_pt=0  float_type=Single  exp_bits=8  fraction_bits=24  quantization=Truncate  overflow=Wrap  en=off  latency=0  dbl_ovrd=off  pipeline=off  block_type=convert
  io_delay : xbsIndex_r4/Delay  rst=off  infoeditControl=Selection of Reset will increase slice count due to use of real FFs and instead of SRLs  en=off  latency=0  dbl_ovrd=off  reg_retiming=on  block_type=delay
  reint1 : xbsIndex_r4/Reinterpret  force_arith_type=on  arith_type=Unsigned  force_bin_pt=on  bin_pt=0  block_type=reinterpret
  sdbe_8_11_network_buffer1_fw_user_data_in : xbsIndex_r4/Gateway Out  inherit_from_input=off  hdl_port=on  timing_constraint=None  locs_specified=off  LOCs={}  UseAsDAC=off  DACChannel='1'  block_type=gatewayout
  sim_out : Outport
  wires:
  io_delay/1 -> cast_gw/1
  cast_gw/1 -> sdbe_8_11_network_buffer1_fw_user_data_in/1
  sdbe_8_11_network_buffer1_fw_user_data_in/1 -> sim_out/1
  out_reg/1 -> assert_reg/1
  assert_reg/1 -> reint1/1
  reint1/1 -> io_delay/1
